simulink model "aerodynamics_comparison"  (R2025b)
settings: Solver=VariableStepAuto  StartTime=0.0  StopTime=10.0  RelTol=1e-3
undefined symbols (not defined in the file): AeroData, Ref_Area, rocket_length, RocketAeroPhysical
libraries: aerolibconvert2 x1
settings Model: Creator=jonno  LastModifiedBy=jonno

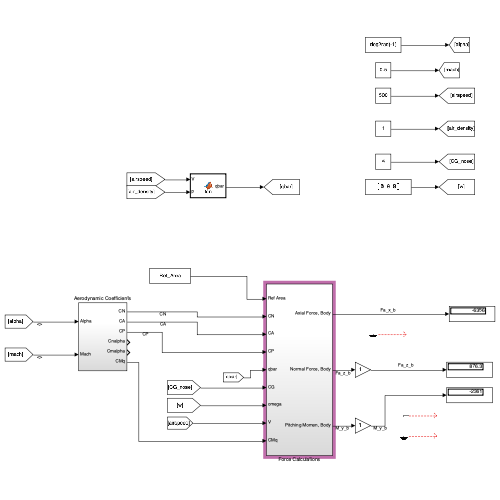
[thumbnail: Simulink's stored preview of the top-level diagram]
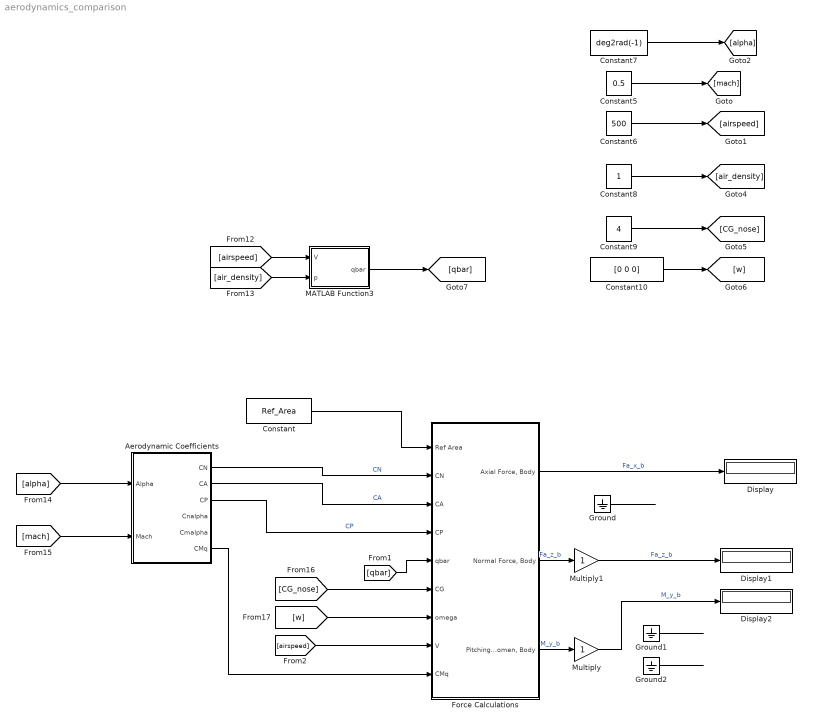
== system aerodynamics_comparison ==
  Aerodynamic Coefficients : Subsystem
  Constant : Constant  Value=Ref_Area  VectorParams1D=off
  Constant10 : Constant  Value=[0 0 0]
  Constant5 : Constant  Value=0.5
  Constant6 : Constant  Value=500
  Constant7 : Constant  Value=deg2rad(-1)
  Constant8 : Constant
  Constant9 : Constant  Value=4
  Display : Display
  Display1 : Display
  Display2 : Display
  Force Calculations : Subsystem
  Ground : Ground
  Ground1 : Ground
  Ground2 : Ground
  MATLAB Function3 : MATLAB Function  TreatAsAtomicUnit=on
  Multiply : Gain
  Multiply1 : Gain
  wires:
  [qbar] -> Force Calculations/5(qbar)
  [w] -> Force Calculations/7(omega)
  [mach] -> Aerodynamic Coefficients/2(Mach)
  [alpha] -> Aerodynamic Coefficients/1(Alpha)
  Multiply1/1 -> Display1/1  "Fa_z_b"
  Multiply/1 -> Display2/1  "M_y_b"
  [CG_nose] -> Force Calculations/6(CG)
  Aerodynamic Coefficients/6(CMq) -> Force Calculations/9(CMq)
  Ground/1 -> ?
  Aerodynamic Coefficients/3(CP) -> Force Calculations/4(CP)  "CP"
  Force Calculations/3("Pitching Momen, Body") -> Multiply/1  "M_y_b"
  Ground2/1 -> ?
  Force Calculations/2("Normal Force, Body") -> Multiply1/1  "Fa_z_b"
  Aerodynamic Coefficients/2(CA) -> Force Calculations/3(CA)  "CA"
  [airspeed] -> Force Calculations/8(V)
  Aerodynamic Coefficients/1(CN) -> Force Calculations/2(CN)  "CN"
  Force Calculations/1("Axial Force, Body") -> Display/1  "Fa_x_b"
  Constant/1 -> Force Calculations/1(Ref Area)
  Ground1/1 -> ?
  Constant5/1 -> [mach]
  Constant6/1 -> [airspeed]
  Constant7/1 -> [alpha]
  Constant8/1 -> [air_density]
  Constant9/1 -> [CG_nose]
  Constant10/1 -> [w]
  [airspeed] -> MATLAB Function3/1(V)
  [air_density] -> MATLAB Function3/2(p)
  MATLAB Function3/1(qbar) -> [qbar]

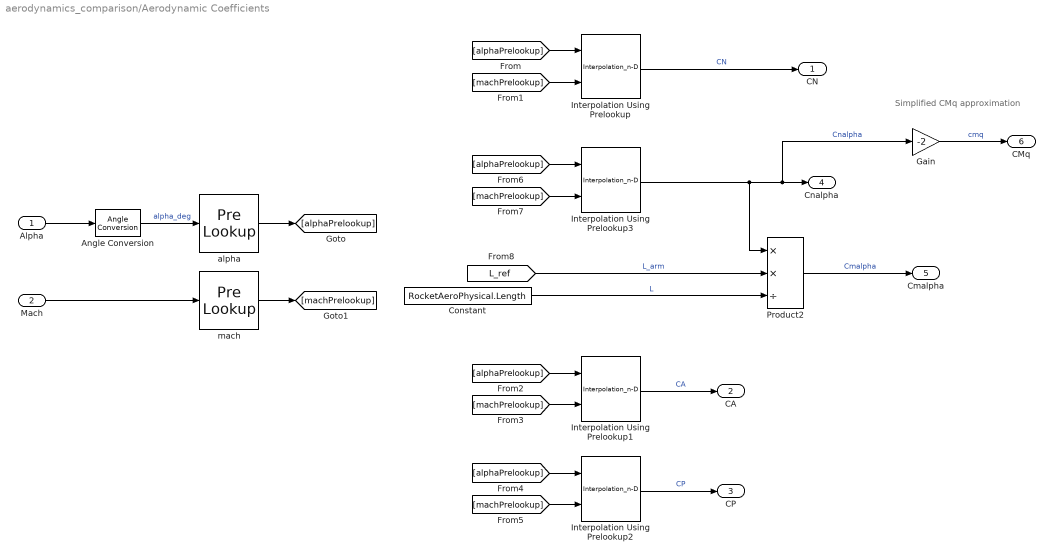
== system aerodynamics_comparison/Aerodynamic Coefficients ==
  note: Simplified CMq approximation
  Alpha : Inport
  Mach : Inport  Port=2
  Angle Conversion : aerolibconvert2/Angle Conversion  IU=rad  OU=deg
  Constant : Constant  Value=RocketAeroPhysical.Length
  Gain : Gain  Gain=-2
  Interpolation Using Prelookup : Interpolation_n-D  Table=AeroData.Tables.CN  RequireIndexFractionAsBus=on  InternalRulePriority=Speed
      settings: InputPortMap=u0,u1
  Interpolation Using Prelookup1 : Interpolation_n-D  Table=AeroData.Tables.CAPower_On  RequireIndexFractionAsBus=on  InternalRulePriority=Speed
      settings: InputPortMap=u0,u1
  Interpolation Using Prelookup2 : Interpolation_n-D  Table=AeroData.Tables.CP  RequireIndexFractionAsBus=on  InternalRulePriority=Speed
      settings: InputPortMap=u0,u1
  Interpolation Using Prelookup3 : Interpolation_n-D  Table=AeroData.Tables.Cnalpha  RequireIndexFractionAsBus=on  InternalRulePriority=Speed
      settings: InputPortMap=u0,u1
  Product2 : Product  Inputs=**/
  alpha : PreLookup  BreakpointsData=AeroData.Breakpoints.Alpha  OutputSelection=Index and fraction as bus  IndexSearchMethod=Evenly spaced points  UseLastBreakpoint=on
  mach : PreLookup  BreakpointsData=AeroData.Breakpoints.Mach  OutputSelection=Index and fraction as bus  IndexSearchMethod=Evenly spaced points  ExtrapMethod=Linear
  CN : Outport
  CA : Outport  Port=2
  CP : Outport  Port=3
  Cnalpha : Outport  Port=4
  Cmalpha : Outport  Port=5
  CMq : Outport  Port=6
  wires:
  Interpolation Using Prelookup/1 -> CN/1  "CN"
  alpha/1 -> [alphaPrelookup]
  mach/1 -> [machPrelookup]
  [alphaPrelookup] -> Interpolation Using Prelookup/1
  [machPrelookup] -> Interpolation Using Prelookup/2
  Interpolation Using Prelookup1/1 -> CA/1  "CA"
  [machPrelookup] -> Interpolation Using Prelookup1/2
  [alphaPrelookup] -> Interpolation Using Prelookup1/1
  Interpolation Using Prelookup2/1 -> CP/1  "CP"
  [machPrelookup] -> Interpolation Using Prelookup2/2
  [alphaPrelookup] -> Interpolation Using Prelookup2/1
  Interpolation Using Prelookup3/1 -> Gain/1, Cnalpha/1, Product2/1  "Cnalpha"
  [machPrelookup] -> Interpolation Using Prelookup3/2
  [alphaPrelookup] -> Interpolation Using Prelookup3/1
  Angle Conversion/1 -> alpha/1  "alpha_deg"
  Mach/1 -> mach/1
  Alpha/1 -> Angle Conversion/1
  [L_ref] -> Product2/2  "L_arm"
  Constant/1 -> Product2/3  "L"
  Product2/1 -> Cmalpha/1  "Cmalpha"
  Gain/1 -> CMq/1  "cmq"

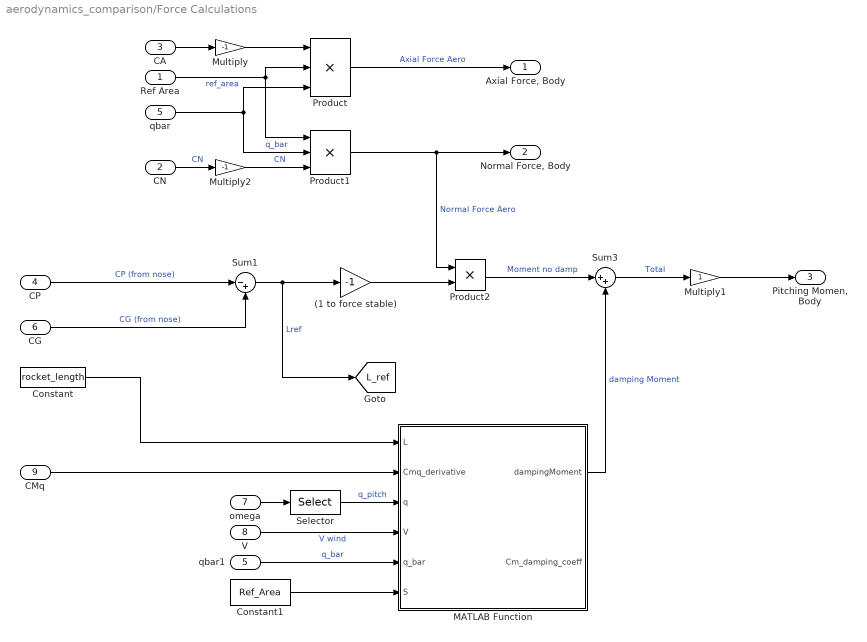
== system aerodynamics_comparison/Force Calculations ==
  Ref Area : Inport
  CN : Inport  Port=2
  CA : Inport  Port=3
  CP : Inport  Port=4
  qbar : Inport  Port=5
  CG : Inport  Port=6
  omega : Inport  Port=7
  V : Inport  Port=8
  CMq : Inport  Port=9
  (1 to force stable) : Gain  Gain=-1
  Constant : Constant  Value=rocket_length
  Constant1 : Constant  Value=Ref_Area
  MATLAB Function : MATLAB Function  TreatAsAtomicUnit=on
  Multiply : Gain  Gain=-1
  Multiply1 : Gain
  Multiply2 : Gain  Gain=-1
  Product : Product  Inputs=***
  Product1 : Product  Inputs=***
  Product2 : Product
  Selector : Selector  InputPortWidth=3  IndexOptions=Index vector (dialog)  Indices=2  OutputSizes=1
  Sum1 : Sum  Inputs=|-+
  Sum3 : Sum  Inputs=|++
  qbar1 : InportShadow  Port=5
  "Axial Force, Body" : Outport
  "Normal Force, Body" : Outport  Port=2
  "Pitching Momen, Body" : Outport  Port=3
  tag scope: L_ref=global
  wires:
  Product/1 -> "Axial Force, Body"/1  "Axial Force Aero"
  CA/1 -> Multiply/1
  qbar/1 -> Product/3, Product1/2  "q_bar"
  Ref Area/1 -> Product/2, Product1/1  "ref_area"
  Multiply/1 -> Product/1
  Multiply2/1 -> Product1/3  "CN"
  CP/1 -> Sum1/1  "CP (from nose)"
  Sum1/1 -> (1 to force stable)/1, [L_ref]  "Lref"
  Product2/1 -> Sum3/1  "Moment no damp"
  Sum3/1 -> Multiply1/1  "Total"
  Constant/1 -> MATLAB Function/1(L)
  Multiply1/1 -> "Pitching Momen, Body"/1
  Product1/1 -> Product2/1, "Normal Force, Body"/1  "Normal Force Aero"
  V/1 -> MATLAB Function/4(V)  "V wind"
  omega/1 -> Selector/1
  Selector/1 -> MATLAB Function/3(q)  "q_pitch"
  qbar1/1 -> MATLAB Function/5(q_bar)  "q_bar"
  CG/1 -> Sum1/2  "CG (from nose)"
  (1 to force stable)/1 -> Product2/2
  Constant1/1 -> MATLAB Function/6(S)
  MATLAB Function/1(dampingMoment) -> Sum3/2  "damping Moment"
  CMq/1 -> MATLAB Function/2(Cmq_derivative)
  CN/1 -> Multiply2/1  "CN"

== matlab function aerodynamics_comparison/MATLAB Function3 ==
  data: V input; qbar output; p input
function qbar = fcn(V, p)



qbar = (1/2)*V^2 * p;

== matlab function aerodynamics_comparison/Force Calculations/MATLAB Function ==
  data: L input; dampingMoment output; Cmq_derivative input; q input; V input; q_bar input; S input; Cm_damping_coeff output
function [dampingMoment, Cm_damping_coeff] = calculateDampingMoment(L, Cmq_derivative, q, V, q_bar, S)
% Calculates the dimensional pitch damping moment from the dimensionless Cmq derivative.
%
% Inputs:
%   L:              Reference length (m)
%   Cmq_derivative: The dimensionless pitch damping derivative (from lookup or approximation)
%   q:              Pitch angular velocity (rad/s)
%   V:              Vehicle velocity (m/s)
%   q_bar:          Dynamic pressure (Pa)
%   S:              Reference area (m^2)
%
% Outputs:
%   dampingMoment:      The final physical damping moment (N*m)
%   Cm_damping_coeff:   The intermediate dimensionless damping moment coefficient

    % Handle the V=0 case to prevent division by zero
    if V == 0
        non_dim_pitch_rate = 0;
    else
        % Calculate the non-dimensional pitch rate (q_hat)
        non_dim_pitch_rate = (q * L) / (2 * V);
    end

    % Calculate the total damping moment coefficient
    Cm_damping_coeff = Cmq_derivative * non_dim_pitch_rate;

    % Convert the coefficient to a physical moment
    dampingMoment = Cm_damping_coeff * q_bar * S * L;

end
